simulink model "Golf_Nonlin_ModaleINOP"  (R2019a)
settings: Solver=VariableStepAuto  StartTime=0.0  StopTime=600  RelTol=1e-3
values from neighbouring files (symbols this model uses):
  alphaTrim = trimVal(2)    [mainProjetCADV_2a.m]
  dPHRTrim = trimVal(1)    [mainProjetCADV_2a.m]
  dthrIdle = 0.1    [mainProjetCADV_2a.m]
  km = trim.kmass(choix)    [utGetTrimPoint.m]
  ms = trim.mStat(choix)    [utGetTrimPoint.m]
  RAD2DEG = 180/pi    (= 57.2957795131)    [mainProjetCADV_2a.m]    (also in utAcDynamicsFunction.m)
  thetaTrim = trimVal(3)    [mainProjetCADV_2a.m]
  uTrim = zeros(TOTAL_CMD, 1)    [mainProjetCADV_2a.m]
  VaTrim = utEas2Tas(Eas_KTS*KTS2MS, hTrimFL*FL2M)    [mainProjetCADV_2a.m]
  xTrim = zeros(TOTAL_SV, 1)    [mainProjetCADV_2a.m]
undefined symbols (not defined in the file or in its folder): A6, aircraftChosen, B6, Cobs, H, K6, Kd, Ki, Kp, L6
settings Model: Creator=bourdiul  LastModifiedBy=mariu

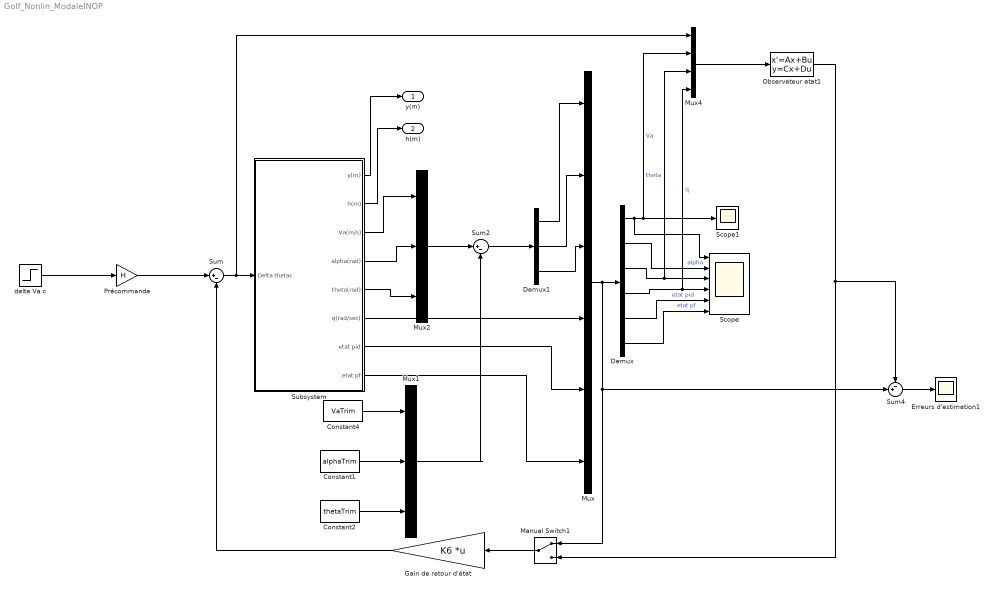
== system Golf_Nonlin_ModaleINOP ==
  Constant1 : Constant  Value=alphaTrim
  Constant2 : Constant  Value=thetaTrim
  Constant4 : Constant  Value=VaTrim
  Demux : Demux  Outputs=6
  Demux1 : Demux  Outputs=3
  Erreurs d'estimation1 : Scope
  Gain de retour d'état : Gain  Gain=K6  Multiplication=Matrix(K*u) (u vector)
  Manual Switch1 : ManualSwitch
  Mux : Mux  Inputs=6
  Mux1 : Mux  Inputs=3
  Mux2 : Mux  Inputs=3
  Mux4 : Mux
  Observateur etat1 : StateSpace  A=A6-L6*Cobs  B=[B6, L6]  C=eye(6)  D=zeros(6,4)  InitialCondition=0
  Précommande : Gain  Gain=H
  Scope : Scope  NumInputPorts=6
  Scope1 : Scope
  Subsystem : Subsystem
  Sum : Sum  Inputs=|+-
  Sum2 : Sum  Inputs=|+-
  Sum4 : Sum  Inputs=-+|
  delta Va c : Step  SampleTime=0
  y(m) : Outport
  h(m) : Outport  Port=2
  wires:
  Demux/5 -> Scope/5  "etat pid"
  Demux1/1 -> Mux/1
  Subsystem/2(h(m)) -> h(m)/1
  Demux1/2 -> Mux/2
  Subsystem/8("etat pf ") -> Mux/6
  Constant2/1 -> Mux1/3
  Demux1/3 -> Mux/3
  Subsystem/7(etat pid) -> Mux/5
  Sum2/1 -> Demux1/1
  Mux1/1 -> Sum2/2
  Constant1/1 -> Mux1/2
  Constant4/1 -> Mux1/1
  Mux2/1 -> Sum2/1
  Subsystem/3(Va(m/s)) -> Mux2/1
  Demux/6 -> Scope/6  "etat pf"
  Demux/4 -> Mux4/4, Scope/4  "q"
  Demux/2 -> Scope/2  "alpha"
  Demux/3 -> Mux4/3, Scope/3  "theta"
  Gain de retour d'état/1 -> Sum/2
  Subsystem/6(q(rad/sec)) -> Mux/4
  Subsystem/5(theta(rad)) -> Mux2/3
  Subsystem/4(alpha(rad)) -> Mux2/2
  Subsystem/1(y(m)) -> y(m)/1
  Sum/1 -> Mux4/1, Subsystem/1("Delta thetac ")
  Demux/1 -> Scope/1, Mux4/2, Scope1/1  "Va"
  delta Va c/1 -> Précommande/1
  Précommande/1 -> Sum/1
  Mux4/1 -> Observateur etat1/1
  Manual Switch1/1 -> Gain de retour d'état/1
  Observateur etat1/1 -> Sum4/1, Manual Switch1/2
  Sum4/1 -> Erreurs d'estimation1/1
  Mux/1 -> Manual Switch1/1, Sum4/2, Demux/1

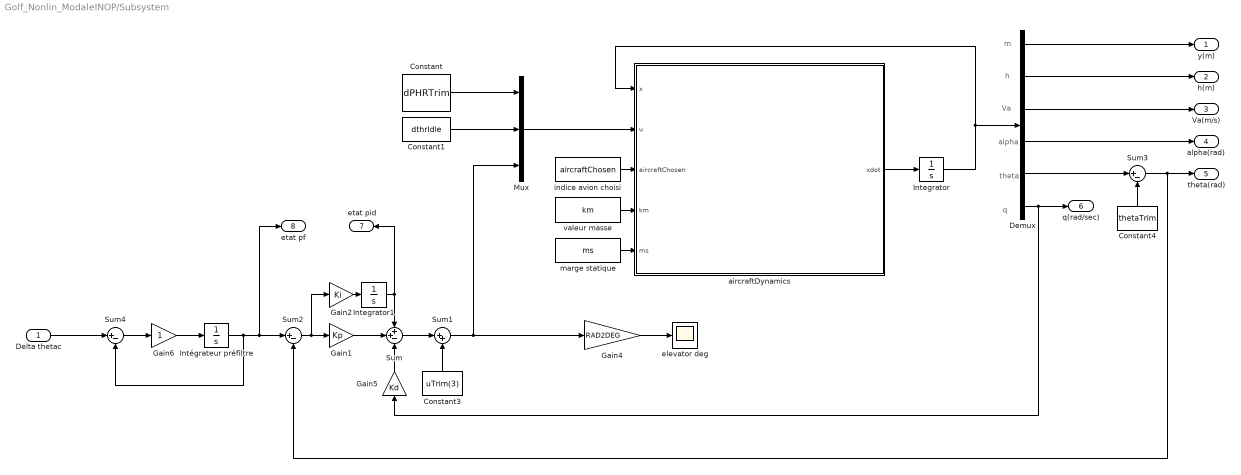
== system Golf_Nonlin_ModaleINOP/Subsystem ==
  note: m
  note: h
  note: Va
  note: alpha
  note: theta
  note: q
  "Delta thetac " : Inport
  Constant : Constant  Value=dPHRTrim
  Constant1 : Constant  Value=dthrIdle
  Constant3 : Constant  Value=uTrim(3)
  Constant4 : Constant  Value=thetaTrim
  Demux : Demux  Outputs=6
  Gain1 : Gain  Gain=Kp
  Gain2 : Gain  Gain=Ki
  Gain4 : Gain  Gain=RAD2DEG
  Gain5 : Gain  Gain=Kd
  Gain6 : Gain
  Integrator : Integrator  InitialCondition=xTrim
  Integrator1 : Integrator
  Intégrateur préfiltre : Integrator
  Mux : Mux  Inputs=3
  Sum : Sum  Inputs=++-
  Sum1 : Sum  Inputs=|++
  Sum2 : Sum  Inputs=|+-
  Sum3 : Sum  Inputs=|+-
  Sum4 : Sum  Inputs=|+-
  aircraftDynamics : MATLAB Function  TreatAsAtomicUnit=on
  elevator deg : Scope
  indice avion choisi : Constant  Value=aircraftChosen
  marge statique : Constant  Value=ms
  valeur masse : Constant  Value=km
  y(m) : Outport
  h(m) : Outport  Port=2
  Va(m/s) : Outport  Port=3
  alpha(rad) : Outport  Port=4
  theta(rad) : Outport  Port=5
  q(rad/sec) : Outport  Port=6
  etat pid : Outport  Port=7
  "etat pf " : Outport  Port=8
  wires:
  aircraftDynamics/1(xdot) -> Integrator/1
  "Delta thetac "/1 -> Sum4/1
  Sum/1 -> Sum1/1
  Sum1/1 -> Mux/3, Gain4/1
  Sum4/1 -> Gain6/1
  Gain2/1 -> Integrator1/1
  Constant/1 -> Mux/1
  Integrator1/1 -> etat pid/1, Sum/1
  Integrator/1 -> aircraftDynamics/1(x), Demux/1
  Demux/6 -> q(rad/sec)/1, Gain5/1
  Demux/1 -> y(m)/1
  Sum2/1 -> Gain2/1, Gain1/1
  Mux/1 -> aircraftDynamics/2(u)
  indice avion choisi/1 -> aircraftDynamics/3(aircraftChosen)
  Demux/3 -> Va(m/s)/1
  Gain4/1 -> elevator deg/1
  marge statique/1 -> aircraftDynamics/5(ms)
  Gain5/1 -> Sum/3
  valeur masse/1 -> aircraftDynamics/4(km)
  Gain1/1 -> Sum/2
  Demux/4 -> alpha(rad)/1
  Constant3/1 -> Sum1/2
  Gain6/1 -> Intégrateur préfiltre/1
  Demux/2 -> h(m)/1
  Intégrateur préfiltre/1 -> "etat pf "/1, Sum2/1, Sum4/2
  Demux/5 -> Sum3/1
  Constant4/1 -> Sum3/2
  Constant1/1 -> Mux/2
  Sum3/1 -> theta(rad)/1, Sum2/2

== matlab function Golf_Nonlin_ModaleINOP/Subsystem/aircraftDynamics ==
  data: x input; u input; xdot output; aircraftChosen input; km input; ms input
function xdot = aircraftDynamics(x,u, aircraftChosen,km,ms)
    TOTAL_SV = 6;
    xIn = zeros(TOTAL_SV,1);
    xIn = x;
    
	TOTAL_CMD = 3;
    uIn = zeros(TOTAL_CMD,1);
    uIn = u;
    
    xdot = utAcDynamicsFunction(xIn,uIn, aircraftChosen,km,ms);
end %aircraftDynamics
